simulink model "GOcontroll_Linux"  (R2023b)
settings: Solver=FixedStepDiscrete  StartTime=0.0  StopTime=5  FixedStep=0.01  RelTol=1e-3
PreLoadFcn:
  | librarySetup
PostLoadFcn:
  | %eval([bdroot,'_startup']) to run model_startup.m
  | Select_Config
  | 
  | core_info = evalc('feature(''numcores'')');
  | core_info_split = split(core_info, " ");
  | num_cores = core_info_split{12};
  | set_param(bdroot, "MakeCommand", ['make_rtw -j' num_cores]);
  | clear num_cores core_info core_info_split
values from neighbouring files (symbols this model uses):
  LEDRed = Simulink.Parameter    [GOcontroll_Linux_startup.m]
libraries: GOcontroll_Moduline_Target x23, etargetslib x6, simulink x3
settings Model: Creator=la_obwlf  LastModifiedBy=maud
settings SolverCC: AlgebraicLoopSolver=TrustRegion
settings DataIOCC: LimitDataPoints=on  SaveFormat=Array  ReturnWorkspaceOutputs=off
settings OptimizationCC: BlockReduction=off  DefaultParameterBehavior=Inlined  LifeSpan=1  EfficientTunableParamExpr=on
settings DebuggingCC: SolverPrmCheckMsg=warning  InheritedTsInSrcMsg=none  MultiTaskRateTransMsg=warning  ParameterPrecisionLossMsg=none  UnconnectedInputMsg=warning  UnconnectedOutputMsg=warning  SFUnusedDataAndEventsDiag=none  SFUnexpectedBacktrackingDiag=warning  SFNoUnconditionalDefaultTransitionDiag=warning  SFUndirectedBroadcastEventsDiag=none  SFExecutionAtInitializationDiag=none  RCSCRenamedMsg=none  RCSCObservableMsg=none  ArithmeticOperatorsInVariantConditions=warning
settings HardwareCC: ProdBitPerLong=64  ProdLargestAtomicInteger=Long  ProdLargestAtomicFloat=Double  ProdLongLongMode=on  ProdHWDeviceType=ARM Compatible->ARM 64-bit (LP64)
settings ModelReferenceCC: EnableRefExpFcnMdlSchedulingChecks=on  PropagateSignalLabelsOutOfModel=off
settings SFSimCC: SimUseLocalCustomCode=off  MATLABDynamicMemAlloc=off  CustomCodeUndefinedFunction=UseInterfaceOnly
settings RTWCC: Description=Linux Embedded Coder  SystemTargetFile=ert_linux.tlc  MakeCommand=make_rtw -j24  TemplateMakefile=ert_linux_target_64.tmf  RetainRTWFile=on  RTWUseLocalCustomCode=off
settings CodeAppCC: IgnoreCustomStorageClasses=off  StateflowObjectComments=on
settings STFCustomTargetCC: TargetLangStandard=C89/C90 (ANSI)  CodeReplacementLibrary=GNU C99 extensions  CombineOutputUpdateFcns=on  ERTCustomFileBanners=on  SupportContinuousTime=off  SupportNonInlinedSFcns=off  RemoveResetFunc=on  MATLABClassNameForMDSCustomization=Simulink.SoftwareTarget.ERTCustomization  SystemTargetFile=ert_linux.tlc
settings ERTTargetCC: CodeReplacementLibrary=GNU C99 extensions  MultiwordLength=2048  ParMdlRefBuildCompliant=off  CompOptLevelCompliant=off  ConcurrentExecutionCompliant=off  ModelStepFunctionPrototypeControlCompliant=off  CPPClassGenCompliant=off  UseToolchainInfoCompliant=off  ERTCustomFileTemplate=ert_linux_file_process.tlc  PreserveExpressionOrder=on  SuppressUnreachableDefaultCases=off
settings ConfigComp: CovMetricSettings=dw  CovSaveCumulativeToWorkspaceVar=on  CovSaveSingleToWorkspaceVar=on  CovExternalEMLEnable=off  CovSFcnEnable=off

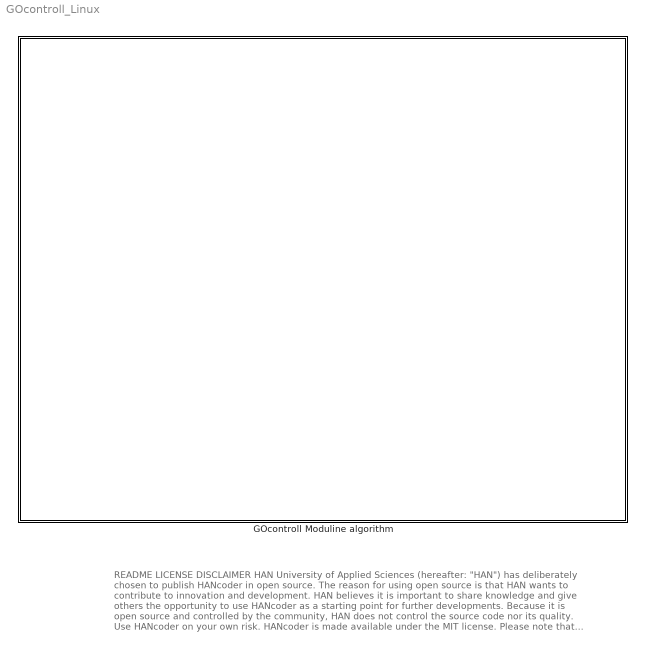
== system GOcontroll_Linux ==
  note: README
      |
      | LICENSE
      |
      | DISCLAIMER
      |
      | HAN University of Applied Sciences (hereafter: "HAN") has deliberately chosen
      | to publish HANcoder in open source. The reason for using open source is that
      | HAN wants to contribute to innovation and development. HAN believes it is
      | important to share knowledge and give others the opportunity to use HANcoder
      | as a starting point for further developments. Because it is open source and
      | controlled by the community, HAN does not control the source code nor its
      | quality. Use HANcoder on your own risk. HANcoder is made available under the
      | MIT license. Please note that this license contains an exclusion of liability.
  GOcontroll Moduline algorithm : Subsystem  mask(TopLevelSubsystem){}
      mask Display: image(imread('GOcontroll.png'))

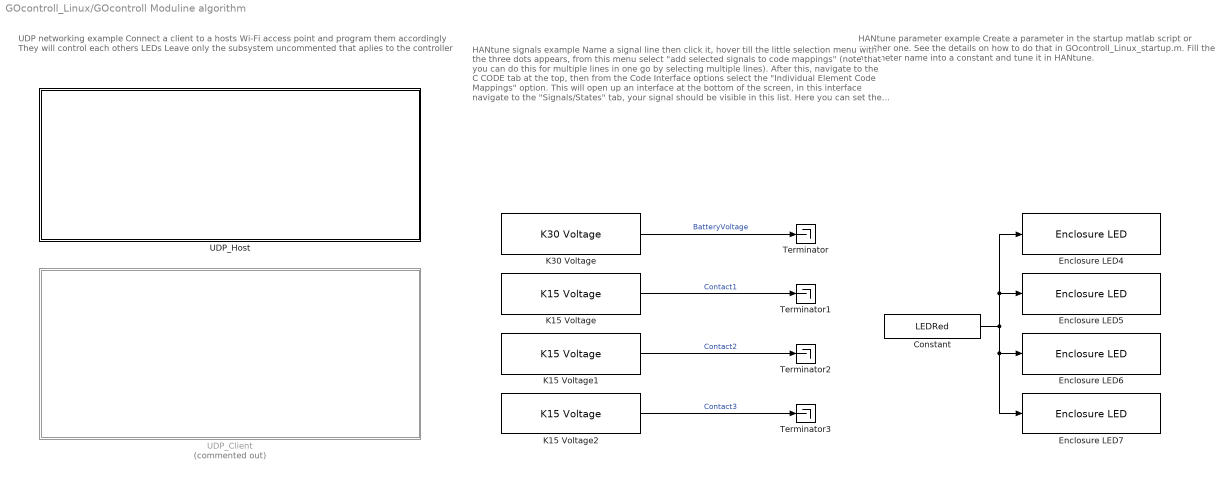
== system GOcontroll_Linux/GOcontroll Moduline algorithm ==
  note: HANtune parameter example
      | Create a parameter in the startup matlab script or another one.
      | See the details on how to do that in GOcontroll_Linux_startup.m.
      | Fill the parameter name into a constant and tune it in HANtune.
  note: HANtune signals example
      | Name a signal line then click it, hover till the little selection menu with
      | the three dots appears, from this menu select "add selected signals
      | to code mappings" (note that you can do this for multiple lines in one go
      | by selecting multiple lines).
      | After this, navigate to the C CODE tab at the top, then from the Code
      | Interface options select the "Individual Element Code Mappings" option.
      | This will open up an interface at the bottom of the screen, in this interface
      | navigate to the "Signals/States" tab, your signal should be visible in this list.
      | Here you can set the storage class to "ExportedGlobal", this can also be
      | done for multiple signals in one go by selecting multiple signals in the list
      | with ctrl or shift click, and then changing the storage class for any of the
      | selected signals.
  note: UDP networking example
      | Connect a client to a hosts Wi-Fi access point and program them accordingly
      | They will control each others LEDs
      | Leave only the subsystem uncommented that aplies to the controller
  Constant : Constant  Value=LEDRed  OutDataTypeStr=uint8
  Enclosure LED4 : GOcontroll_Moduline_Target/Enclosure LED's/Enclosure LED  Tag=HANcoder_GOcontroll_Moduline_IV  tsamp=-1  led=1  color=Red
      settings: SourceProductName=GOcontroll Moduline
  Enclosure LED5 : GOcontroll_Moduline_Target/Enclosure LED's/Enclosure LED  Tag=HANcoder_GOcontroll_Moduline_IV  tsamp=-1  led=2  color=Red
      settings: SourceProductName=GOcontroll Moduline
  Enclosure LED6 : GOcontroll_Moduline_Target/Enclosure LED's/Enclosure LED  Tag=HANcoder_GOcontroll_Moduline_IV  tsamp=-1  led=3  color=Red
      settings: SourceProductName=GOcontroll Moduline
  Enclosure LED7 : GOcontroll_Moduline_Target/Enclosure LED's/Enclosure LED  Tag=HANcoder_GOcontroll_Moduline_IV  tsamp=-1  led=4  color=Red
      settings: SourceProductName=GOcontroll Moduline
  K15 Voltage : GOcontroll_Moduline_Target/Supply control/K15 Voltage  Tag=HANcoder_GOcontroll_Moduline_IV  ContrType=GOcontroll Moduline IV  tsamp=0.1  k15pin=K15-1 (Connector C pin 2)
      settings: SourceProductName=GOcontroll Moduline
  K15 Voltage1 : GOcontroll_Moduline_Target/Supply control/K15 Voltage  Tag=HANcoder_GOcontroll_Moduline_IV  ContrType=GOcontroll Moduline IV  tsamp=0.1  k15pin=K15-2 (Connector C pin 3)
      settings: SourceProductName=GOcontroll Moduline
  K15 Voltage2 : GOcontroll_Moduline_Target/Supply control/K15 Voltage  Tag=HANcoder_GOcontroll_Moduline_IV  ContrType=GOcontroll Moduline IV  tsamp=0.1  k15pin=K15-3 (Connector C pin 4)
      settings: SourceProductName=GOcontroll Moduline
  K30 Voltage : GOcontroll_Moduline_Target/Supply control/K30 Voltage  Tag=HANcoder_GOcontroll_Moduline_IV  ContrType=GOcontroll Moduline IV  tsamp=0.1
      settings: SourceProductName=GOcontroll Moduline
  Terminator{,1..3} (4 alike) : Terminator
  UDP_Client : Subsystem  Commented=on
  UDP_Host : Subsystem
  wires:
  Constant/1 -> Enclosure LED7/1, Enclosure LED6/1, Enclosure LED4/1, Enclosure LED5/1
  K15 Voltage/1 -> Terminator1/1  "Contact1"
  K15 Voltage2/1 -> Terminator3/1  "Contact3"
  K30 Voltage/1 -> Terminator/1  "BatteryVoltage"
  K15 Voltage1/1 -> Terminator2/1  "Contact2"

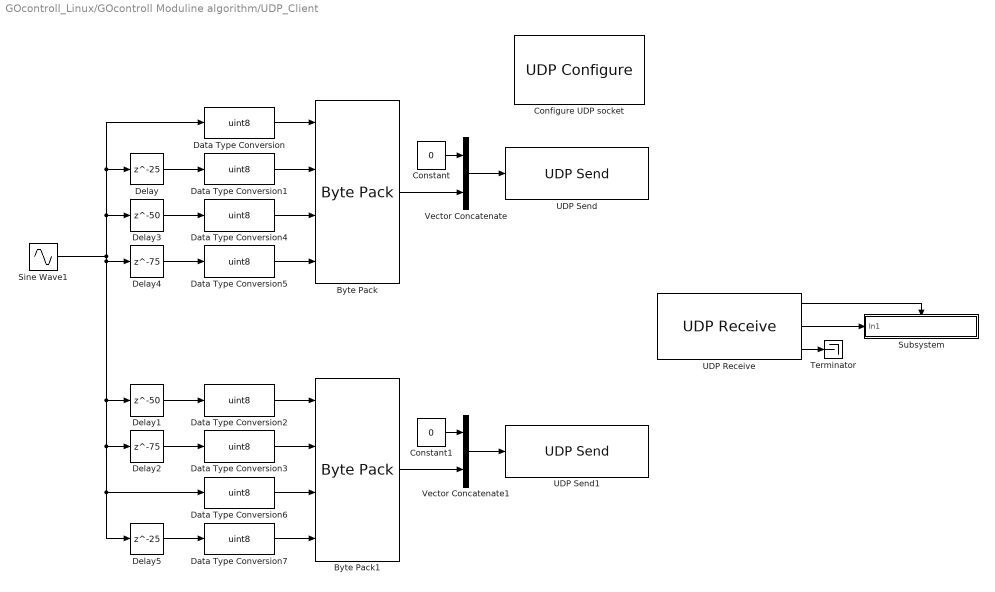
== system GOcontroll_Linux/GOcontroll Moduline algorithm/UDP_Client ==
  Byte Pack : etargetslib/Byte Pack  datatypes=SineWaveTypes  byteAlign=1
  Byte Pack1 : etargetslib/Byte Pack  datatypes=SineWaveTypes  byteAlign=1
  Configure UDP socket : GOcontroll_Moduline_Target/Network/UDP/UDP Configure  socket_id=id  port=9001  ip='0.0.0.0'  broadcast=on
      settings: SourceProductName=GOcontroll Moduline
  Constant : Constant  Value=0  OutDataTypeStr=uint8
  Constant1 : Constant  Value=0  OutDataTypeStr=uint8
  Data Type Conversion{,1..7} (8 alike) : DataTypeConversion  OutDataTypeStr=uint8  SaturateOnIntegerOverflow=off  RndMeth=Floor
  Delay : Delay  DelayLength=25
  Delay1 : Delay  DelayLength=50
  Delay2 : Delay  DelayLength=75
  Delay3 : Delay  DelayLength=50
  Delay4 : Delay  DelayLength=75
  Delay5 : Delay  DelayLength=25
  Sine Wave1 : Sin  SineType=Sample based  Amplitude=120  Bias=121  Phase=128  Samples=100  SampleTime=0.01
  Subsystem : Subsystem
  Terminator : Terminator
  UDP Receive : GOcontroll_Moduline_Target/Network/UDP/UDP Receive  tsamp=-1  socket_id=id  buff_len=UDPBuffSize
      settings: SourceProductName=GOcontroll Moduline
  UDP Send : GOcontroll_Moduline_Target/Network/UDP/UDP Send  socket_id=<empty>  ip='192.168.19.85'  port=9000  tsamp=0.01
      settings: SourceProductName=GOcontroll Moduline
  UDP Send1 : GOcontroll_Moduline_Target/Network/UDP/UDP Send  socket_id=<empty>  ip='192.168.19.85'  port=9000  tsamp=0.01
      settings: SourceProductName=GOcontroll Moduline
  Vector Concatenate : Concatenate
  Vector Concatenate1 : Concatenate
  wires:
  Data Type Conversion/1 -> Byte Pack/1
  Delay/1 -> Data Type Conversion1/1
  Byte Pack/1 -> Vector Concatenate/2
  Data Type Conversion3/1 -> Byte Pack1/2
  Delay1/1 -> Data Type Conversion2/1
  Data Type Conversion1/1 -> Byte Pack/2
  Delay2/1 -> Data Type Conversion3/1
  Data Type Conversion2/1 -> Byte Pack1/1
  Byte Pack1/1 -> Vector Concatenate1/2
  Delay4/1 -> Data Type Conversion5/1
  Delay3/1 -> Data Type Conversion4/1
  Data Type Conversion5/1 -> Byte Pack/4
  Data Type Conversion4/1 -> Byte Pack/3
  Sine Wave1/1 -> Delay3/1, Data Type Conversion/1, Delay/1, Delay4/1, Data Type Conversion6/1, Delay5/1, Delay2/1, Delay1/1
  Delay5/1 -> Data Type Conversion7/1
  Data Type Conversion7/1 -> Byte Pack1/4
  Data Type Conversion6/1 -> Byte Pack1/3
  UDP Receive/3 -> Terminator/1
  UDP Receive/2 -> Subsystem/1(In1)
  UDP Receive/1 -> Subsystem/Trigger
  Vector Concatenate/1 -> UDP Send/1
  Constant/1 -> Vector Concatenate/1
  Vector Concatenate1/1 -> UDP Send1/1
  Constant1/1 -> Vector Concatenate1/1

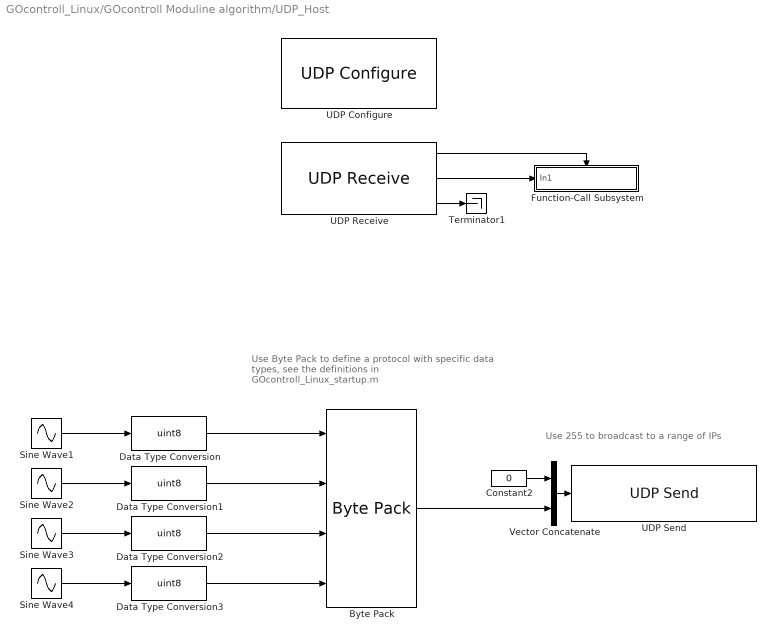
== system GOcontroll_Linux/GOcontroll Moduline algorithm/UDP_Host ==
  note: Use 255 to broadcast to a range of IPs
  note: Use Byte Pack to define a protocol with
      | specific data types, see the definitions in
      | GOcontroll_Linux_startup.m
  Byte Pack : etargetslib/Byte Pack  datatypes=SineWaveTypes  byteAlign=1
  Constant2 : Constant  Value=0  OutDataTypeStr=uint8
  Data Type Conversion{,1..3} (4 alike) : DataTypeConversion  OutDataTypeStr=uint8  SaturateOnIntegerOverflow=off  RndMeth=Floor
  Function-Call Subsystem : Subsystem  TreatAsAtomicUnit=on
  Sine Wave{1..4} (4 alike) : Sin  SineType=Sample based  Amplitude=120  Bias=121  Phase=128  Samples=100  SampleTime=0.01
  Terminator1 : Terminator
  UDP Configure : GOcontroll_Moduline_Target/Network/UDP/UDP Configure  socket_id=led_sinus  port=9000  ip='0.0.0.0'  broadcast=on
      settings: SourceProductName=GOcontroll Moduline
  UDP Receive : GOcontroll_Moduline_Target/Network/UDP/UDP Receive  tsamp=-1  socket_id=led_sinus  buff_len=UDPBuffSize
      settings: SourceProductName=GOcontroll Moduline
  UDP Send : GOcontroll_Moduline_Target/Network/UDP/UDP Send  socket_id=led_sinus  ip='192.168.255.255'  port=9001  tsamp=0.01
      settings: SourceProductName=GOcontroll Moduline
  Vector Concatenate : Concatenate
  wires:
  Data Type Conversion2/1 -> Byte Pack/3
  Data Type Conversion/1 -> Byte Pack/1
  Sine Wave3/1 -> Data Type Conversion2/1
  Data Type Conversion3/1 -> Byte Pack/4
  Byte Pack/1 -> Vector Concatenate/2
  Data Type Conversion1/1 -> Byte Pack/2
  Sine Wave2/1 -> Data Type Conversion1/1
  Constant2/1 -> Vector Concatenate/1
  Sine Wave1/1 -> Data Type Conversion/1
  Sine Wave4/1 -> Data Type Conversion3/1
  UDP Receive/1 -> Function-Call Subsystem/Trigger
  UDP Receive/2 -> Function-Call Subsystem/1(In1)
  UDP Receive/3 -> Terminator1/1
  Vector Concatenate/1 -> UDP Send/1

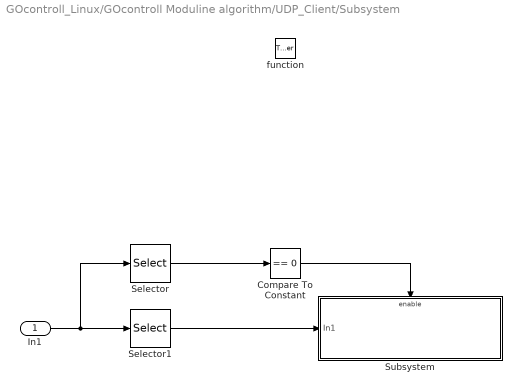
== system GOcontroll_Linux/GOcontroll Moduline algorithm/UDP_Client/Subsystem ==
  In1 : Inport
  function : TriggerPort  TriggerType=function-call  VariantControl=(inherit)
  Compare To Constant : simulink/Logic and Bit Operations/Compare To Constant  relop===  const=0  OutDataTypeStr=boolean
  Selector : Selector  IndexMode=Zero-based  InputPortWidth=5  IndexOptions=Index vector (dialog)  Indices=[0]  OutputSizes=1
  Selector1 : Selector  IndexMode=Zero-based  InputPortWidth=5  IndexOptions=Starting index (dialog)  Indices=[1]  OutputSizes=4
  Subsystem : Subsystem
  wires:
  In1/1 -> Selector1/1, Selector/1
  Selector/1 -> Compare To Constant/1
  Compare To Constant/1 -> Subsystem/Enable
  Selector1/1 -> Subsystem/1(In1)

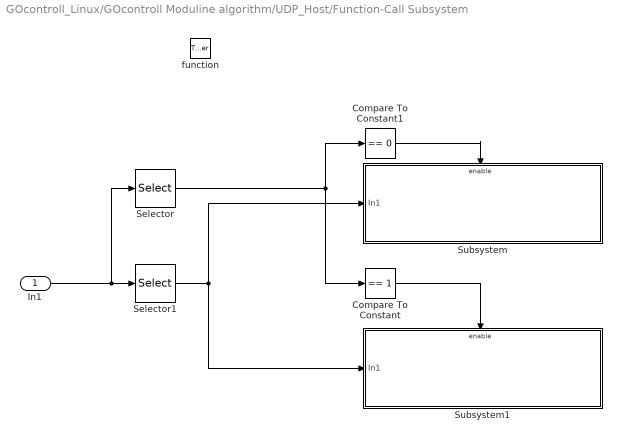
== system GOcontroll_Linux/GOcontroll Moduline algorithm/UDP_Host/Function-Call Subsystem ==
  In1 : Inport
  function : TriggerPort  TriggerType=function-call  VariantControl=(inherit)
  Compare To Constant : simulink/Logic and Bit Operations/Compare To Constant  relop===  const=1  OutDataTypeStr=boolean
  Compare To Constant1 : simulink/Logic and Bit Operations/Compare To Constant  relop===  const=0  OutDataTypeStr=boolean
  Selector : Selector  IndexMode=Zero-based  InputPortWidth=5  IndexOptions=Index vector (dialog)  Indices=[0]  OutputSizes=1
  Selector1 : Selector  IndexMode=Zero-based  InputPortWidth=5  IndexOptions=Starting index (dialog)  Indices=[1]  OutputSizes=4
  Subsystem : Subsystem
  Subsystem1 : Subsystem
  wires:
  In1/1 -> Selector1/1, Selector/1
  Selector/1 -> Compare To Constant/1, Compare To Constant1/1
  Compare To Constant/1 -> Subsystem1/Enable
  Compare To Constant1/1 -> Subsystem/Enable
  Selector1/1 -> Subsystem/1(In1), Subsystem1/1(In1)

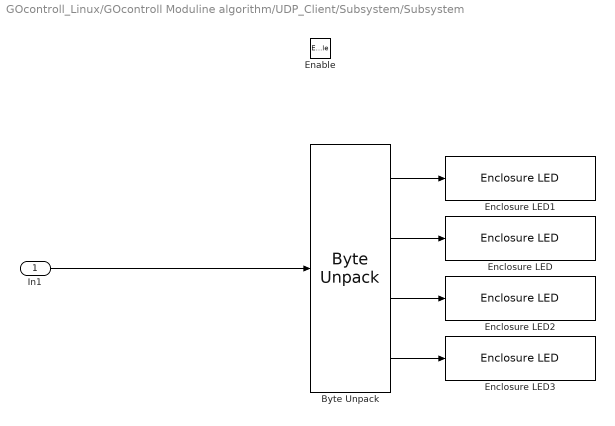
== system GOcontroll_Linux/GOcontroll Moduline algorithm/UDP_Client/Subsystem/Subsystem ==
  In1 : Inport
  Enable : EnablePort
  Byte Unpack : etargetslib/Byte Unpack  dimensions=SineWaveSizes  datatypes=SineWaveTypes  byteAlign=1
  Enclosure LED : GOcontroll_Moduline_Target/Enclosure LED's/Enclosure LED  Tag=HANcoder_TARGET_STM32_Olimexino  led=2  color=Blue
      settings: SourceProductName=GOcontroll Moduline
  Enclosure LED1 : GOcontroll_Moduline_Target/Enclosure LED's/Enclosure LED  Tag=HANcoder_TARGET_STM32_Olimexino  led=1  color=Blue
      settings: SourceProductName=GOcontroll Moduline
  Enclosure LED2 : GOcontroll_Moduline_Target/Enclosure LED's/Enclosure LED  Tag=HANcoder_TARGET_STM32_Olimexino  led=3  color=Blue
      settings: SourceProductName=GOcontroll Moduline
  Enclosure LED3 : GOcontroll_Moduline_Target/Enclosure LED's/Enclosure LED  Tag=HANcoder_TARGET_STM32_Olimexino  led=4  color=Blue
      settings: SourceProductName=GOcontroll Moduline
  wires:
  Byte Unpack/4 -> Enclosure LED3/1
  In1/1 -> Byte Unpack/1
  Byte Unpack/1 -> Enclosure LED1/1
  Byte Unpack/2 -> Enclosure LED/1
  Byte Unpack/3 -> Enclosure LED2/1

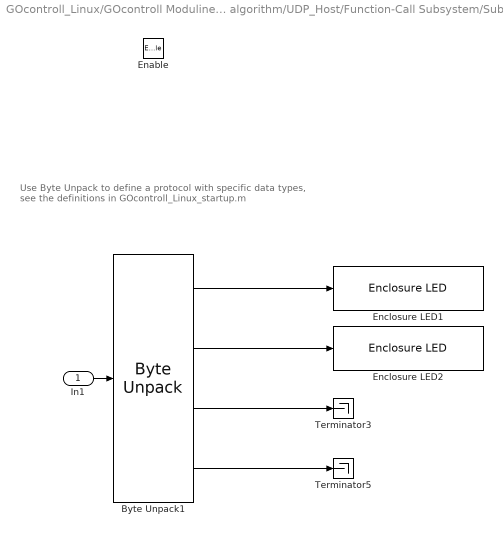
== system GOcontroll_Linux/GOcontroll Moduline algorithm/UDP_Host/Function-Call Subsystem/Subsystem ==
  note: Use Byte Unpack to define a protocol with
      | specific data types, see the definitions in
      | GOcontroll_Linux_startup.m
  In1 : Inport
  Enable : EnablePort
  Byte Unpack1 : etargetslib/Byte Unpack  dimensions=SineWaveSizes  datatypes=SineWaveTypes  byteAlign=1
  Enclosure LED1 : GOcontroll_Moduline_Target/Enclosure LED's/Enclosure LED  Tag=HANcoder_TARGET_STM32_Olimexino  tsamp=-1  led=1  color=Blue
      settings: SourceProductName=GOcontroll Moduline
  Enclosure LED2 : GOcontroll_Moduline_Target/Enclosure LED's/Enclosure LED  Tag=HANcoder_TARGET_STM32_Olimexino  tsamp=-1  led=3  color=Blue
      settings: SourceProductName=GOcontroll Moduline
  Terminator3 : Terminator
  Terminator5 : Terminator
  wires:
  Byte Unpack1/4 -> Terminator5/1
  Byte Unpack1/3 -> Terminator3/1
  Byte Unpack1/1 -> Enclosure LED1/1
  Byte Unpack1/2 -> Enclosure LED2/1
  In1/1 -> Byte Unpack1/1

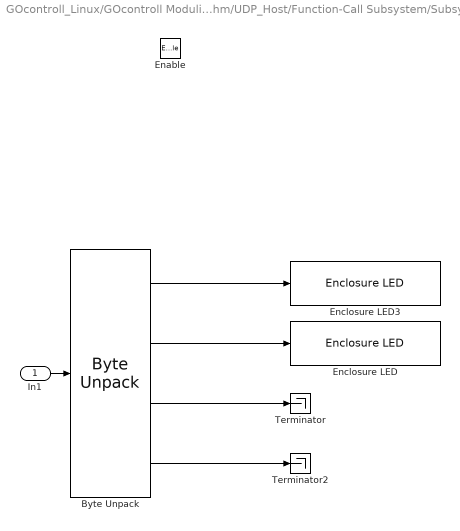
== system GOcontroll_Linux/GOcontroll Moduline algorithm/UDP_Host/Function-Call Subsystem/Subsystem1 ==
  In1 : Inport
  Enable : EnablePort
  Byte Unpack : etargetslib/Byte Unpack  dimensions=SineWaveSizes  datatypes=SineWaveTypes  byteAlign=1
  Enclosure LED : GOcontroll_Moduline_Target/Enclosure LED's/Enclosure LED  Tag=HANcoder_TARGET_STM32_Olimexino  tsamp=-1  led=2  color=Blue
      settings: SourceProductName=GOcontroll Moduline
  Enclosure LED3 : GOcontroll_Moduline_Target/Enclosure LED's/Enclosure LED  Tag=HANcoder_TARGET_STM32_Olimexino  tsamp=-1  led=4  color=Blue
      settings: SourceProductName=GOcontroll Moduline
  Terminator : Terminator
  Terminator2 : Terminator
  wires:
  Byte Unpack/1 -> Enclosure LED3/1
  Byte Unpack/2 -> Enclosure LED/1
  Byte Unpack/3 -> Terminator/1
  In1/1 -> Byte Unpack/1
  Byte Unpack/4 -> Terminator2/1
